simulink model "CmdParModeGlissant"  (R2019b)
settings: Solver=VariableStepAuto  StartTime=0.0  StopTime=100  RelTol=1e-3
values from neighbouring files (symbols this model uses):
  c = 0.5    [CommandeParModeGlissant.m]    (also in SimulinkData.mat)
  km = 1    [CommandeParModeGlissant.m]    (also in SimulinkData.mat)
  m = 2    [CommandeParModeGlissant.m]    (also in SimulinkData.mat)
settings Model: Creator=PC  LastModifiedBy=PC
settings SolverCC: ZeroCrossAlgorithm=Adaptive
settings DebuggingCC: IgnoredZcDiagnostic=none

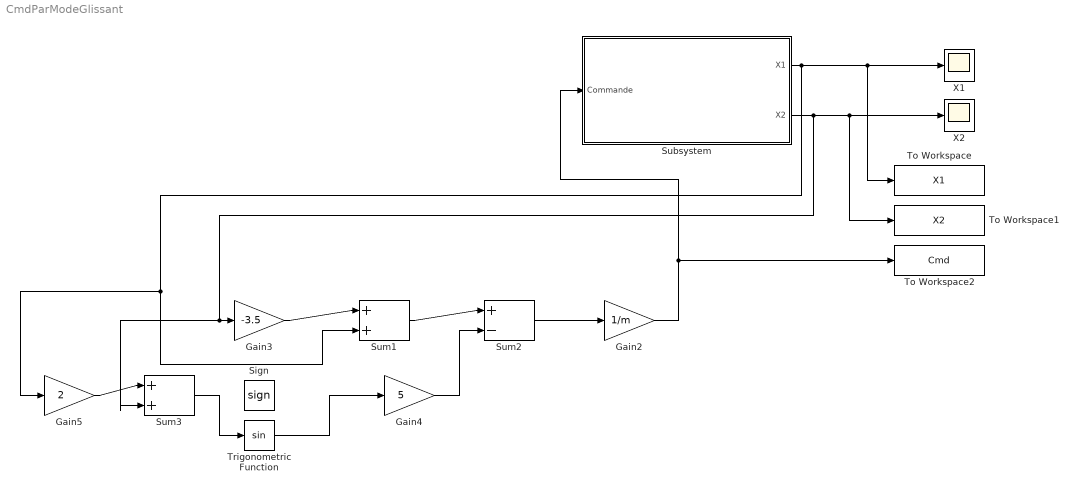
== system CmdParModeGlissant ==
  Gain2 : Gain  Gain=1/m
  Gain3 : Gain  Gain=-3.5
  Gain4 : Gain  Gain=5
  Gain5 : Gain  Gain=2
  Sign : Signum
  Subsystem : Subsystem
  Sum1 : Sum  Inputs=|++
  Sum2 : Sum  Inputs=|+-
  Sum3 : Sum  Inputs=|++
  To Workspace : ToWorkspace  VariableName=X1  SaveFormat=Timeseries  SampleTime=-1
  To Workspace1 : ToWorkspace  VariableName=X2  SaveFormat=Timeseries  SampleTime=-1
  To Workspace2 : ToWorkspace  VariableName=Cmd  SaveFormat=Timeseries  SampleTime=-1
  Trigonometric Function : Trigonometry
  X1 : Scope
  X2 : Scope
  wires:
  Gain3/1 -> Sum1/1
  Sum1/1 -> Sum2/1
  Sum2/1 -> Gain2/1
  Gain4/1 -> Sum2/2
  Trigonometric Function/1 -> Gain4/1
  Gain5/1 -> Sum3/1
  Sum3/1 -> Trigonometric Function/1
  Subsystem/1(X1) -> Gain5/1, Sum1/2, To Workspace/1, X1/1
  Subsystem/2(X2) -> Sum3/2, Gain3/1, To Workspace1/1, X2/1
  Gain2/1 -> To Workspace2/1, Subsystem/1("Commande ")

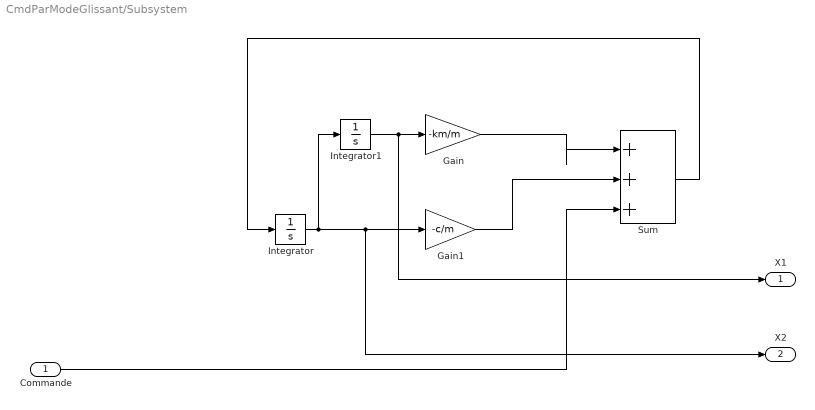
== system CmdParModeGlissant/Subsystem ==
  "Commande " : Inport
  Gain : Gain  Gain=-km/m
  Gain1 : Gain  Gain=-c/m
  Integrator : Integrator
  Integrator1 : Integrator  InitialCondition=1
  Sum : Sum  Inputs=|+++
  X1 : Outport
  X2 : Outport  Port=2
  wires:
  Gain1/1 -> Sum/2
  Sum/1 -> Integrator/1
  Integrator1/1 -> X1/1, Gain/1
  "Commande "/1 -> Sum/3
  Gain/1 -> Sum/1
  Integrator/1 -> X2/1, Gain1/1, Integrator1/1
